simulink model "Powertrain_model_SEV_21b"  (R2021b)
settings: Solver=VariableStepAuto  StartTime=0.0  StopTime=tspan  RelTol=1e-3
values from neighbouring files (symbols this model uses):
  bsfc_idle_GE = 4.96e03    (= 4960)    [Sim_script.m]
  DR = 5.213    [Sim_script.m]
  drawn_pow_M = 464.6018    [Sim_script.m]
  Gensetdata = Gensetdata1    [Sim_script.m]
  motor_eff = motor_eff_PMSM    [Sim_script.m]
  Trans_In = 24.086    [Sim_script.m]
  tspan = 10800    [Sim_script.m]
  w_CE_idle = 400    [Sim_script.m]
undefined symbols (not defined in the file or in its folder): dailyloadl, eta_EM_map, resT_conv_bollard, resT_conv_free, resT_conv_tow, T_EM_col, T_EM_max, w_EM_row
libraries: slpidlib x1
settings Model: Creator=user  LastModifiedBy=olsonsao

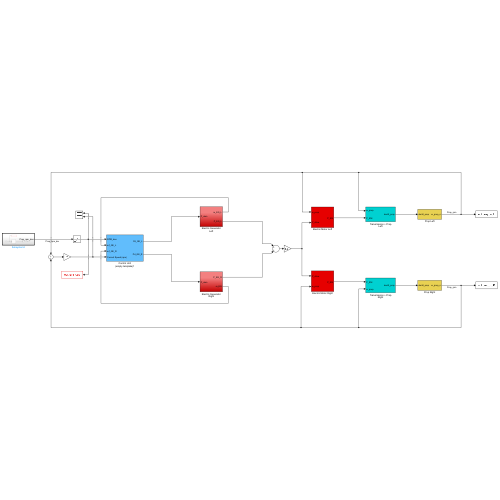
[thumbnail: Simulink's stored preview of the top-level diagram]
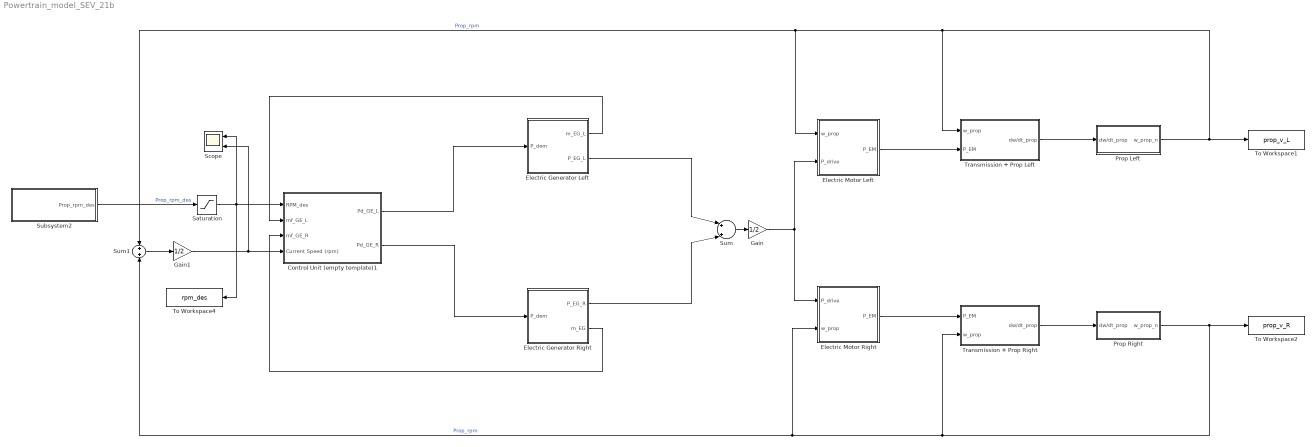
== system Powertrain_model_SEV_21b ==
  Control Unit (empty template)1 : Subsystem  Tag=control unit
  Electric Generator Left : Subsystem
  Electric Generator Right : Subsystem
  Electric Motor Left : Subsystem
  Electric Motor Right : Subsystem
  Gain : Gain  Gain=1/2
  Gain1 : Gain  Gain=1/2
  Prop Left : Subsystem
  Prop Right : Subsystem
  Saturation : Saturate  UpperLimit=inf  LowerLimit=w_CE_idle/DR
  Scope : Scope  NumInputPorts=2
  Subsystem2 : Subsystem  TreatAsAtomicUnit=on
  Sum : Sum  Inputs=|+|+|
  Sum1 : Sum  Inputs=+|+
  To Workspace1 : ToWorkspace  VariableName=prop_v_L  SampleTime=-1
      settings: Save2DSignal=2-D array (concatenate along first dimension)
  To Workspace2 : ToWorkspace  VariableName=prop_v_R  SampleTime=-1
      settings: Save2DSignal=2-D array (concatenate along first dimension)
  To Workspace4 : ToWorkspace  VariableName=rpm_des  SampleTime=-1
      settings: Save2DSignal=2-D array (concatenate along first dimension)
  Transmission + Prop Left : Subsystem
  Transmission + Prop Right : Subsystem
  wires:
  Sum/1 -> Gain/1
  Gain/1 -> Electric Motor Right/1(P_drive), Electric Motor Left/2(P_drive)
  Electric Motor Left/1(P_EM) -> Transmission + Prop Left/2(P_EM)
  Prop Left/1(w_prop_n) -> To Workspace1/1, Transmission + Prop Left/1(w_prop), Electric Motor Left/1(w_prop), Sum1/1  "Prop_rpm"
  Electric Motor Right/1(P_EM) -> Transmission + Prop Right/1(P_EM)
  Prop Right/1(w_prop_n) -> Transmission + Prop Right/2(w_prop), Electric Motor Right/2(w_prop), Sum1/2, To Workspace2/1  "Prop_rpm"
  Gain1/1 -> Scope/2, Control Unit (empty template)1/4(Current Speed (rpm))
  Subsystem2/1(Prop_rpm_des) -> Saturation/1  "Prop_rpm_des"
  Electric Generator Left/1(m_EG_L) -> Control Unit (empty template)1/2(mf_GE_L)
  Electric Generator Right/2(m_EG) -> Control Unit (empty template)1/3(mf_GE_R)
  Sum1/1 -> Gain1/1
  Transmission + Prop Left/1(dw/dt_prop) -> Prop Left/1(dw/dt_prop)
  Transmission + Prop Right/1(dw/dt_prop) -> Prop Right/1(dw/dt_prop)
  Control Unit (empty template)1/2(Pd_GE_R) -> Electric Generator Right/1(P_dem)
  Electric Generator Right/1(P_EG_R) -> Sum/2
  Control Unit (empty template)1/1(Pd_GE_L) -> Electric Generator Left/1(P_dem)
  Electric Generator Left/2(P_EG_L) -> Sum/1
  Saturation/1 -> Control Unit (empty template)1/1(RPM_des), To Workspace4/1, Scope/1

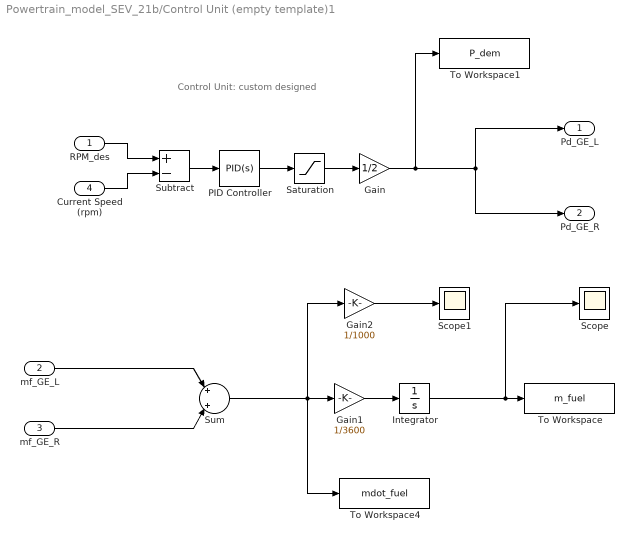
== system Powertrain_model_SEV_21b/Control Unit (empty template)1 ==
  note: Control Unit: custom designed
  RPM_des : Inport
  mf_GE_L : Inport  Port=2
  mf_GE_R : Inport  Port=3
  Current Speed (rpm) : Inport  Port=4
  Gain : Gain  Gain=1/2
  Gain1 : Gain  Gain=1/3600
  Gain2 : Gain  Gain=1/1000
  Integrator : Integrator
  PID Controller : slpidlib/PID Controller  Controller=PID  Form=Parallel  TimeDomain=Continuous-time  UseExternalTs=off  SampleTime=-1  IntegratorMethod=Forward Euler  FilterMethod=Forward Euler  ControllerParametersSource=internal  P=1.27731937948155  I=0.314602230470785  D=0.413734700213223  UseFilter=on  N=0.624884340967824  TunerSelectOption=Transfer Function Based (PID Tuner App)  InitialConditionSource=internal  InitialConditionForIntegrator=0  InitialConditionForFilter=0  DifferentiatorICPrevScaledInput=0  ExternalReset=none  TrackingMode=off  Kt=1  LimitOutput=on  SatLimitsSource=internal  UpperSaturationLimit=inf  LowerSaturationLimit=0  LinearizeAsGain=on  AntiWindupMode=none  Kb=1  POutMin=[]  POutMax=[]  IOutMin=[]  IOutMax=[]  DOutMin=[]  DOutMax=[]  NOutMin=[]  NOutMax=[]  SumOutMin=[]  SumOutMax=[]  SaturationOutMin=[]  SaturationOutMax=[]  PParamMin=[]  PParamMax=[]  IParamMin=[]  IParamMax=[]  DParamMin=[]  DParamMax=[]  NParamMin=[]  NParamMax=[]  KbParamMin=[]  KbParamMax=[]  KtParamMin=[]  KtParamMax=[]  KbOutMin=[]  KbOutMax=[]  KtOutMin=[]  KtOutMax=[]  IntegratorOutMin=[]  IntegratorOutMax=[]  FilterOutMin=[]  FilterOutMax=[]  SumI1OutMin=[]  SumI1OutMax=[]  SumI2OutMin=[]  SumI2OutMax=[]  SumI3OutMin=[]  SumI3OutMax=[]  SumI4OutMin=[]  SumI4OutMax=[]  SumDOutMin=[]  SumDOutMax=[]  DifferentiatorOutMin=[]  DifferentiatorOutMax=[]  FilterDiffOutCoefMin=[]  FilterDiffOutCoefMax=[]  ReciprocalOutMin=[]  ReciprocalOutMax=[]  SumDenOutMin=[]  SumDenOutMax=[]  SumNumOutMin=[]  SumNumOutMax=[]  DivideOutMin=[]  DivideOutMax=[]  UdiffTsProdOutMin=[]  UdiffTsProdOutMax=[]  NTsProdOutMin=[]  NTsProdOutMax=[]  UintegralTsProdOutMin=[]  UintegralTsProdOutMax=[]  UngainTsProdOutMin=[]  UngainTsProdOutMax=[]  IntegratorContinuousStateAttributes=''  IntegratorStateMustResolveToSignalObject=off  IntegratorRTWStateStorageClass=Auto  FilterContinuousStateAttributes=''  FilterStateMustResolveToSignalObject=off  FilterRTWStateStorageClass=Auto  ParallelPVariant=InternalParameters  IdealPVariant=Disabled  IVariant=InternalParameters  DVariant=InternalParameters  IntegratorVariant=Continuous  SatVariant=Enabled  AWVariant=Passthrough  PCopyVariant=Disabled  TRVariant=Disabled  FdbkBlocksVariant=Forward  IdealPFdbkVariant=Disabled  SatFdbkVariant=Disabled  DerivativeFilterVariant=ContFilter  NVariant=InternalParameters  NCopyVariant=Disabled  FilterICVariant=InternalICsFilter  IntegratorICVariant=InternalICs  ExternalResetVariant=Disabled  TRSumVariant=Passthrough  SumFdbkVariant=Disabled  SumVariant=Sum_PID  TsampFilterVariant=InternalTs  TsampNgainVariant=Passthrough  TsampIntegralVariant=Passthrough  ExternalSaturationOutDataTypeStr=Inherit: Same as second input
  Saturation : Saturate  UpperLimit=inf  LowerLimit=0
  Scope : Scope
  Scope1 : Scope
  Subtract : Sum  Inputs=+-
  Sum : Sum  Inputs=|+|+|
  To Workspace : ToWorkspace  VariableName=m_fuel  SampleTime=-1
      settings: Save2DSignal=2-D array (concatenate along first dimension)
  To Workspace1 : ToWorkspace  VariableName=P_dem  SampleTime=-1
      settings: Save2DSignal=2-D array (concatenate along first dimension)
  To Workspace4 : ToWorkspace  VariableName=mdot_fuel  SampleTime=-1
      settings: Save2DSignal=2-D array (concatenate along first dimension)
  Pd_GE_L : Outport  InitialOutput=0
  Pd_GE_R : Outport  Port=2  InitialOutput=0
  wires:
  Current Speed (rpm)/1 -> Subtract/2
  RPM_des/1 -> Subtract/1
  Subtract/1 -> PID Controller/1
  mf_GE_L/1 -> Sum/1
  mf_GE_R/1 -> Sum/2
  PID Controller/1 -> Saturation/1
  Saturation/1 -> Gain/1
  Gain/1 -> To Workspace1/1, Pd_GE_R/1, Pd_GE_L/1
  Gain1/1 -> Integrator/1
  Integrator/1 -> To Workspace/1, Scope/1
  Gain2/1 -> Scope1/1
  Sum/1 -> To Workspace4/1, Gain2/1, Gain1/1

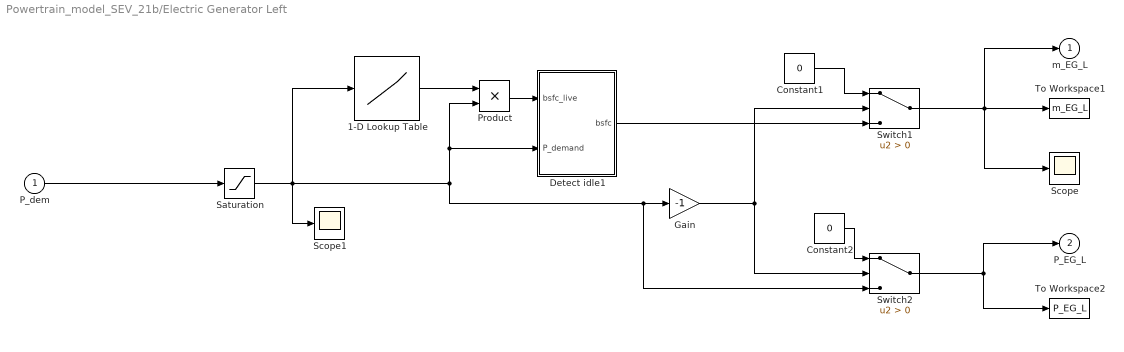
== system Powertrain_model_SEV_21b/Electric Generator Left ==
  P_dem : Inport
  1-D Lookup Table : Lookup_n-D  NumberOfTableDimensions=1  BreakpointsForDimension1=Gensetdata.('Power(kW)')  Table=Gensetdata.('Bsfc(g/kWh)')  InterpMethod=Cubic spline  ExtrapMethod=Cubic spline  InternalRulePriority=Speed  RndMeth=Simplest  InputSameDT=on
  Constant1 : Constant  Value=0
  Constant2 : Constant  Value=0
  Detect idle1 : Subsystem
  Gain : Gain  Gain=-1
  Product : Product
  Saturation : Saturate  UpperLimit=2500  LowerLimit=0
  Scope : Scope
  Scope1 : Scope
  Switch1 : Switch  Criteria=u2 > Threshold
  Switch2 : Switch  Criteria=u2 > Threshold
  To Workspace1 : ToWorkspace  VariableName=m_EG_L  SampleTime=-1
      settings: Save2DSignal=2-D array (concatenate along first dimension)
  To Workspace2 : ToWorkspace  VariableName=P_EG_L  SampleTime=-1
      settings: Save2DSignal=2-D array (concatenate along first dimension)
  m_EG_L : Outport  InitialOutput=0
  P_EG_L : Outport  Port=2  InitialOutput=0
  wires:
  1-D Lookup Table/1 -> Product/1
  Saturation/1 -> Scope1/1, Switch2/3, Gain/1, Detect idle1/2(P_demand), Product/2, 1-D Lookup Table/1
  P_dem/1 -> Saturation/1
  Product/1 -> Detect idle1/1(bsfc_live)
  Gain/1 -> Switch1/2, Switch2/2
  Constant1/1 -> Switch1/1
  Constant2/1 -> Switch2/1
  Detect idle1/1(bsfc) -> Switch1/3
  Switch1/1 -> Scope/1, To Workspace1/1, m_EG_L/1
  Switch2/1 -> To Workspace2/1, P_EG_L/1

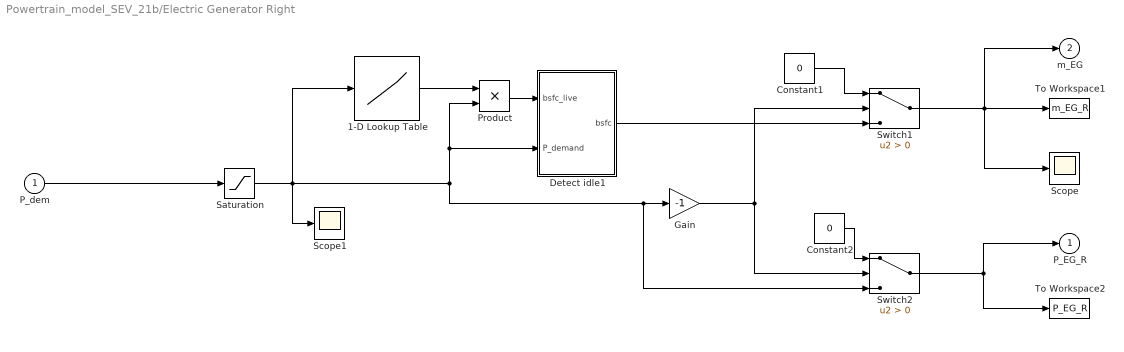
== system Powertrain_model_SEV_21b/Electric Generator Right ==
  P_dem : Inport
  1-D Lookup Table : Lookup_n-D  NumberOfTableDimensions=1  BreakpointsForDimension1=Gensetdata.('Power(kW)')  Table=Gensetdata.('Bsfc(g/kWh)')  InterpMethod=Cubic spline  ExtrapMethod=Cubic spline  InternalRulePriority=Speed  RndMeth=Simplest  InputSameDT=on
  Constant1 : Constant  Value=0
  Constant2 : Constant  Value=0
  Detect idle1 : Subsystem
  Gain : Gain  Gain=-1
  Product : Product
  Saturation : Saturate  UpperLimit=2500  LowerLimit=0
  Scope : Scope
  Scope1 : Scope
  Switch1 : Switch  Criteria=u2 > Threshold
  Switch2 : Switch  Criteria=u2 > Threshold
  To Workspace1 : ToWorkspace  VariableName=m_EG_R  SampleTime=-1
      settings: Save2DSignal=2-D array (concatenate along first dimension)
  To Workspace2 : ToWorkspace  VariableName=P_EG_R  SampleTime=-1
      settings: Save2DSignal=2-D array (concatenate along first dimension)
  P_EG_R : Outport  InitialOutput=0
  m_EG : Outport  Port=2  InitialOutput=0
  wires:
  1-D Lookup Table/1 -> Product/1
  Saturation/1 -> Scope1/1, Switch2/3, Gain/1, Detect idle1/2(P_demand), Product/2, 1-D Lookup Table/1
  P_dem/1 -> Saturation/1
  Product/1 -> Detect idle1/1(bsfc_live)
  Gain/1 -> Switch1/2, Switch2/2
  Constant1/1 -> Switch1/1
  Constant2/1 -> Switch2/1
  Detect idle1/1(bsfc) -> Switch1/3
  Switch1/1 -> Scope/1, To Workspace1/1, m_EG/1
  Switch2/1 -> To Workspace2/1, P_EG_R/1

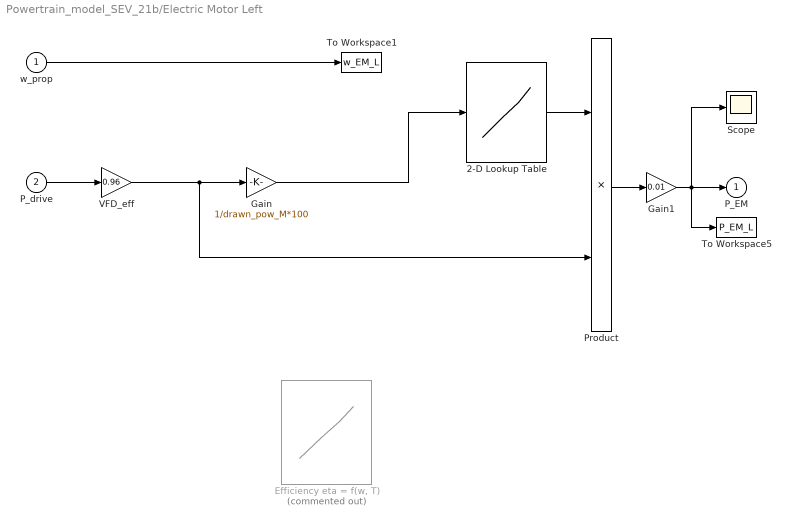
== system Powertrain_model_SEV_21b/Electric Motor Left ==
  w_prop : Inport
  P_drive : Inport  Port=2
  2-D Lookup Table : Lookup_n-D  NumberOfTableDimensions=1  BreakpointsForDimension1=motor_eff.('%power')  BreakpointsForDimension2=T_EM_col  Table=motor_eff.('eff')  InterpMethod=Cubic spline  ExtrapMethod=Cubic spline  InternalRulePriority=Speed  RndMeth=Simplest  InputSameDT=on
  "Efficiency eta = f(w, T)" : Lookup2D  Commented=on  RowIndex=w_EM_row  ColumnIndex=T_EM_col  Table=eta_EM_map
  Gain : Gain  Gain=1/drawn_pow_M*100
  Gain1 : Gain  Gain=0.01
  Product : Product  InputSameDT=on  RndMeth=Zero  SaturateOnIntegerOverflow=on  OutDataTypeStr=Inherit: Same as first input
  Scope : Scope
  To Workspace1 : ToWorkspace  VariableName=w_EM_L  SampleTime=-1
      settings: Save2DSignal=2-D array (concatenate along first dimension)
  To Workspace5 : ToWorkspace  VariableName=P_EM_L  SampleTime=-1
      settings: Save2DSignal=2-D array (concatenate along first dimension)
  VFD_eff : Gain  Gain=0.96
  P_EM : Outport  InitialOutput=0
  wires:
  Product/1 -> Gain1/1
  P_drive/1 -> VFD_eff/1
  2-D Lookup Table/1 -> Product/1
  w_prop/1 -> To Workspace1/1
  Gain/1 -> 2-D Lookup Table/1
  VFD_eff/1 -> Gain/1, Product/2
  Gain1/1 -> Scope/1, To Workspace5/1, P_EM/1

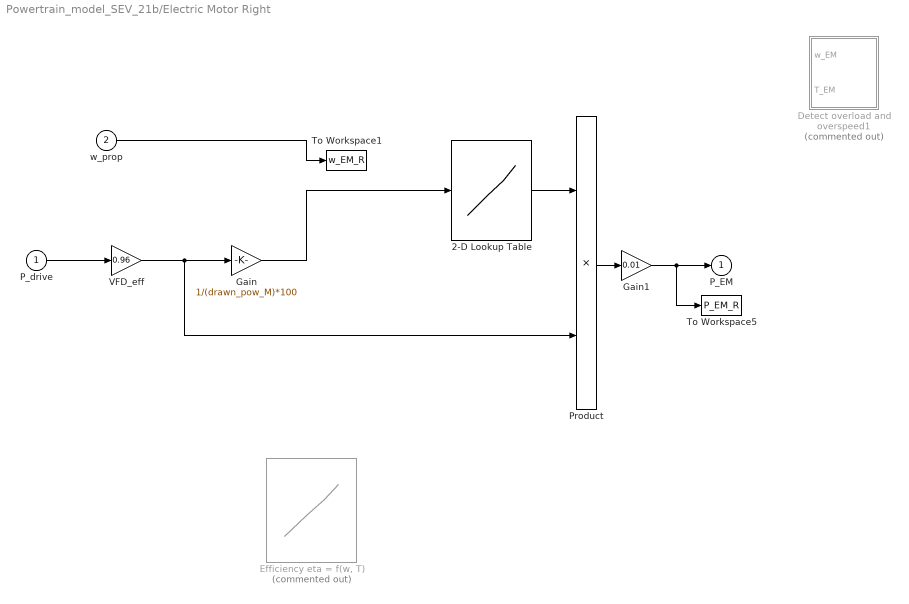
== system Powertrain_model_SEV_21b/Electric Motor Right ==
  P_drive : Inport
  w_prop : Inport  Port=2
  2-D Lookup Table : Lookup_n-D  NumberOfTableDimensions=1  BreakpointsForDimension1=motor_eff.('%power')  BreakpointsForDimension2=T_EM_col  Table=motor_eff.('eff')  InterpMethod=Cubic spline  ExtrapMethod=Cubic spline  InternalRulePriority=Speed  RndMeth=Simplest  InputSameDT=on
  Detect overload and overspeed1 : Subsystem  Commented=on
  "Efficiency eta = f(w, T)" : Lookup2D  Commented=on  RowIndex=w_EM_row  ColumnIndex=T_EM_col  Table=eta_EM_map
  Gain : Gain  Gain=1/(drawn_pow_M)*100
  Gain1 : Gain  Gain=0.01
  Product : Product  InputSameDT=on  RndMeth=Zero  SaturateOnIntegerOverflow=on  OutDataTypeStr=Inherit: Same as first input
  To Workspace1 : ToWorkspace  VariableName=w_EM_R  SampleTime=-1
      settings: Save2DSignal=2-D array (concatenate along first dimension)
  To Workspace5 : ToWorkspace  VariableName=P_EM_R  SampleTime=-1
      settings: Save2DSignal=2-D array (concatenate along first dimension)
  VFD_eff : Gain  Gain=0.96
  P_EM : Outport  InitialOutput=0
  wires:
  Product/1 -> Gain1/1
  P_drive/1 -> VFD_eff/1
  2-D Lookup Table/1 -> Product/1
  w_prop/1 -> To Workspace1/1
  Gain/1 -> 2-D Lookup Table/1
  VFD_eff/1 -> Gain/1, Product/2
  Gain1/1 -> To Workspace5/1, P_EM/1

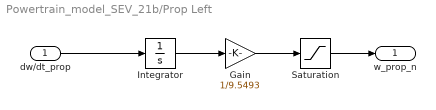
== system Powertrain_model_SEV_21b/Prop Left ==
  dw/dt_prop : Inport
  Gain : Gain  Gain=1/9.5493
  Integrator : Integrator  InitialCondition=w_CE_idle/DR  LowerSaturationLimit=1
  Saturation : Saturate  UpperLimit=inf  LowerLimit=0
  w_prop_n : Outport
  wires:
  dw/dt_prop/1 -> Integrator/1
  Integrator/1 -> Gain/1
  Saturation/1 -> w_prop_n/1
  Gain/1 -> Saturation/1

== system Powertrain_model_SEV_21b/Prop Right ==
  dw/dt_prop : Inport
  Gain : Gain  Gain=1/9.5493
  Integrator : Integrator  InitialCondition=w_CE_idle/DR  LowerSaturationLimit=1
  Saturation : Saturate  UpperLimit=inf  LowerLimit=0
  w_prop_n : Outport
  wires:
  dw/dt_prop/1 -> Integrator/1
  Integrator/1 -> Gain/1
  Saturation/1 -> w_prop_n/1
  Gain/1 -> Saturation/1

== system Powertrain_model_SEV_21b/Subsystem2 ==
  1-D Lookup Table : Lookup_n-D  NumberOfTableDimensions=1  BreakpointsForDimension1=[1:10800]  Table=dailyloadl.('m_sec')  InternalRulePriority=Speed  RndMeth=Simplest  InputSameDT=on
  Clock : Clock
  Gain : Gain
  To Workspace3 : ToWorkspace  VariableName=t  SampleTime=-1
      settings: Save2DSignal=2-D array (concatenate along first dimension)
  Prop_rpm_des : Outport
  wires:
  Clock/1 -> To Workspace3/1, 1-D Lookup Table/1
  1-D Lookup Table/1 -> Gain/1
  Gain/1 -> Prop_rpm_des/1

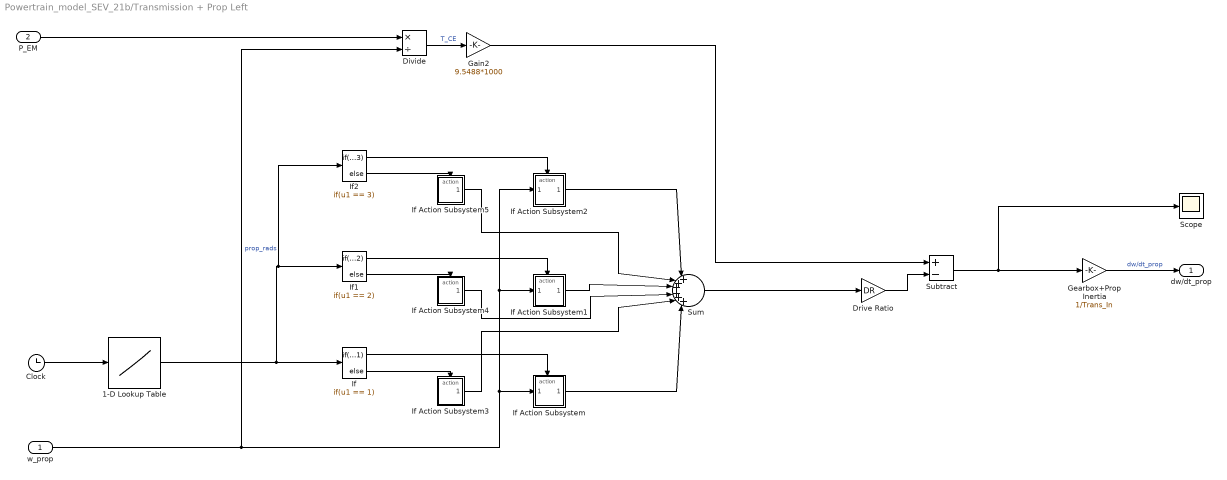
== system Powertrain_model_SEV_21b/Transmission + Prop Left ==
  w_prop : Inport
  P_EM : Inport  Port=2
  1-D Lookup Table : Lookup_n-D  NumberOfTableDimensions=1  BreakpointsForDimension1=[1:tspan]  Table=dailyloadl.('m_mode')  InternalRulePriority=Speed  RndMeth=Simplest  InputSameDT=on
  Clock : Clock
  Divide : Product  Inputs=*/
  Drive Ratio : Gain  Gain=DR
  Gain2 : Gain  Gain=9.5488*1000
  Gearbox+Prop Inertia : Gain  Gain=1/Trans_In
  If : If  IfExpression=u1 == 1
  If Action Subsystem : Subsystem  TreatAsAtomicUnit=on
  If Action Subsystem1 : Subsystem  TreatAsAtomicUnit=on
  If Action Subsystem2 : Subsystem  TreatAsAtomicUnit=on
  If Action Subsystem3 : Subsystem  TreatAsAtomicUnit=on
  If Action Subsystem4 : Subsystem  TreatAsAtomicUnit=on
  If Action Subsystem5 : Subsystem  TreatAsAtomicUnit=on
  If1 : If  IfExpression=u1 == 2
  If2 : If  IfExpression=u1 == 3
  Scope : Scope
  Subtract : Sum  Inputs=+-
  Sum : Sum  Inputs=|++++++|
  dw/dt_prop : Outport
  wires:
  P_EM/1 -> Divide/1
  Gearbox+Prop Inertia/1 -> dw/dt_prop/1  "dw/dt_prop"
  Subtract/1 -> Gearbox+Prop Inertia/1, Scope/1
  Divide/1 -> Gain2/1  "T_CE"
  Gain2/1 -> Subtract/1
  w_prop/1 -> If Action Subsystem2/1(w_prop), If Action Subsystem1/1(w_prop), If Action Subsystem/1(w_prop), Divide/2  "prop_rads"
  Drive Ratio/1 -> Subtract/2
  1-D Lookup Table/1 -> If2/1, If1/1, If/1
  Clock/1 -> 1-D Lookup Table/1
  If/1 -> If Action Subsystem/Action
  If/2 -> If Action Subsystem3/Action
  If1/1 -> If Action Subsystem1/Action
  If2/1 -> If Action Subsystem2/Action
  If2/2 -> If Action Subsystem5/Action
  If1/2 -> If Action Subsystem4/Action
  If Action Subsystem2/1(Out1) -> Sum/1
  If Action Subsystem5/1(Out1) -> Sum/2
  If Action Subsystem/1(Out1) -> Sum/6
  If Action Subsystem3/1(Out1) -> Sum/5
  If Action Subsystem1/1(Out1) -> Sum/3
  If Action Subsystem4/1(Out1) -> Sum/4
  Sum/1 -> Drive Ratio/1

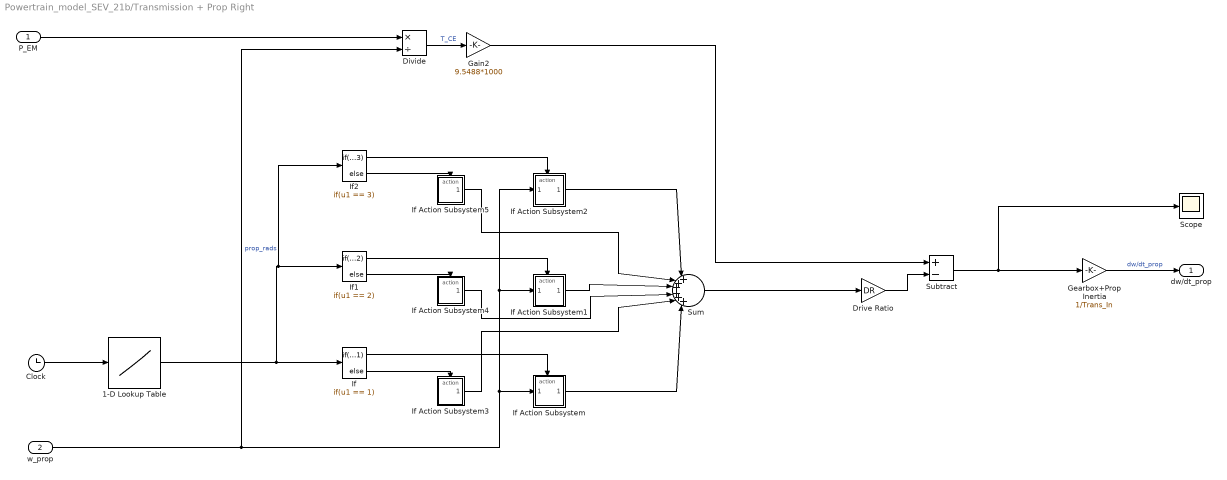
== system Powertrain_model_SEV_21b/Transmission + Prop Right ==
  P_EM : Inport
  w_prop : Inport  Port=2
  1-D Lookup Table : Lookup_n-D  NumberOfTableDimensions=1  BreakpointsForDimension1=[1:tspan]  Table=dailyloadl.('m_mode')  InternalRulePriority=Speed  RndMeth=Simplest  InputSameDT=on
  Clock : Clock
  Divide : Product  Inputs=*/
  Drive Ratio : Gain  Gain=DR
  Gain2 : Gain  Gain=9.5488*1000
  Gearbox+Prop Inertia : Gain  Gain=1/Trans_In
  If : If  IfExpression=u1 == 1
  If Action Subsystem : Subsystem  TreatAsAtomicUnit=on
  If Action Subsystem1 : Subsystem  TreatAsAtomicUnit=on
  If Action Subsystem2 : Subsystem  TreatAsAtomicUnit=on
  If Action Subsystem3 : Subsystem  TreatAsAtomicUnit=on
  If Action Subsystem4 : Subsystem  TreatAsAtomicUnit=on
  If Action Subsystem5 : Subsystem  TreatAsAtomicUnit=on
  If1 : If  IfExpression=u1 == 2
  If2 : If  IfExpression=u1 == 3
  Scope : Scope
  Subtract : Sum  Inputs=+-
  Sum : Sum  Inputs=|++++++|
  dw/dt_prop : Outport
  wires:
  P_EM/1 -> Divide/1
  Gearbox+Prop Inertia/1 -> dw/dt_prop/1  "dw/dt_prop"
  Subtract/1 -> Gearbox+Prop Inertia/1, Scope/1
  Divide/1 -> Gain2/1  "T_CE"
  Gain2/1 -> Subtract/1
  w_prop/1 -> If Action Subsystem2/1(w_prop), If Action Subsystem1/1(w_prop), If Action Subsystem/1(w_prop), Divide/2  "prop_rads"
  Drive Ratio/1 -> Subtract/2
  1-D Lookup Table/1 -> If2/1, If1/1, If/1
  Clock/1 -> 1-D Lookup Table/1
  If/1 -> If Action Subsystem/Action
  If/2 -> If Action Subsystem3/Action
  If1/1 -> If Action Subsystem1/Action
  If2/1 -> If Action Subsystem2/Action
  If2/2 -> If Action Subsystem5/Action
  If1/2 -> If Action Subsystem4/Action
  If Action Subsystem2/1(Out1) -> Sum/1
  If Action Subsystem5/1(Out1) -> Sum/2
  If Action Subsystem/1(Out1) -> Sum/6
  If Action Subsystem3/1(Out1) -> Sum/5
  If Action Subsystem1/1(Out1) -> Sum/3
  If Action Subsystem4/1(Out1) -> Sum/4
  Sum/1 -> Drive Ratio/1

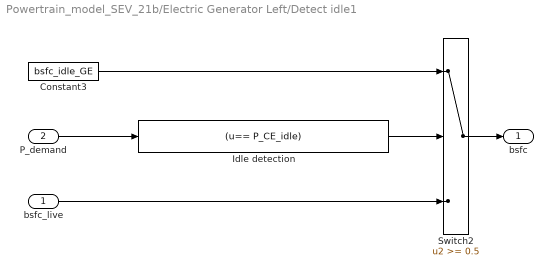
== system Powertrain_model_SEV_21b/Electric Generator Left/Detect idle1 ==
  bsfc_live : Inport
  P_demand : Inport  Port=2
  Constant3 : Constant  Value=bsfc_idle_GE
  Idle detection : Fcn  Expr=(u== P_CE_idle)
  Switch2 : Switch  Threshold=0.5  SaturateOnIntegerOverflow=on  InputSameDT=on
  bsfc : Outport  InitialOutput=0
  wires:
  P_demand/1 -> Idle detection/1
  Idle detection/1 -> Switch2/2
  bsfc_live/1 -> Switch2/3
  Switch2/1 -> bsfc/1
  Constant3/1 -> Switch2/1

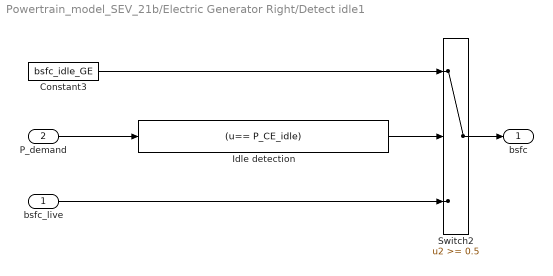
== system Powertrain_model_SEV_21b/Electric Generator Right/Detect idle1 ==
  bsfc_live : Inport
  P_demand : Inport  Port=2
  Constant3 : Constant  Value=bsfc_idle_GE
  Idle detection : Fcn  Expr=(u== P_CE_idle)
  Switch2 : Switch  Threshold=0.5  SaturateOnIntegerOverflow=on  InputSameDT=on
  bsfc : Outport  InitialOutput=0
  wires:
  P_demand/1 -> Idle detection/1
  Idle detection/1 -> Switch2/2
  bsfc_live/1 -> Switch2/3
  Switch2/1 -> bsfc/1
  Constant3/1 -> Switch2/1

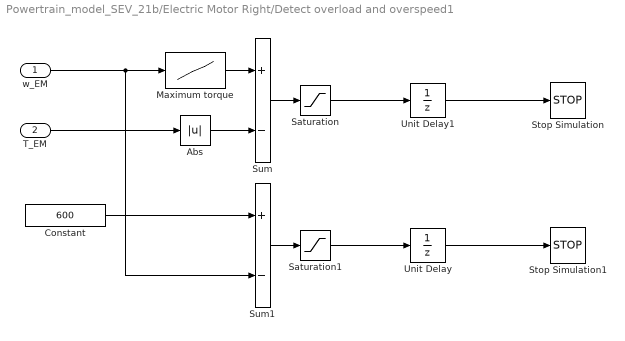
== system Powertrain_model_SEV_21b/Electric Motor Right/Detect overload and overspeed1 ==
  w_EM : Inport
  T_EM : Inport  Port=2
  Abs : Abs  SaturateOnIntegerOverflow=on
  Constant : Constant  Value=600
  Maximum torque : Lookup  InputValues=w_EM_row  Table=T_EM_max  SaturateOnIntegerOverflow=on
  Saturation : Saturate  UpperLimit=0  LowerLimit=-inf
  Saturation1 : Saturate  UpperLimit=0  LowerLimit=-inf
  Stop Simulation : Stop
  Stop Simulation1 : Stop
  Sum : Sum  Inputs=+-  InputSameDT=on  SaturateOnIntegerOverflow=on  OutDataTypeStr=Inherit: Same as first input
  Sum1 : Sum  Inputs=+-  InputSameDT=on  SaturateOnIntegerOverflow=on  OutDataTypeStr=Inherit: Same as first input
  Unit Delay : UnitDelay  SampleTime=-1  HasFrameUpgradeWarning=on
  Unit Delay1 : UnitDelay  SampleTime=-1  HasFrameUpgradeWarning=on
  wires:
  Saturation1/1 -> Unit Delay/1
  Sum1/1 -> Saturation1/1
  Constant/1 -> Sum1/1
  Saturation/1 -> Unit Delay1/1
  Abs/1 -> Sum/2
  Maximum torque/1 -> Sum/1
  T_EM/1 -> Abs/1
  w_EM/1 -> Sum1/2, Maximum torque/1
  Sum/1 -> Saturation/1
  Unit Delay/1 -> Stop Simulation1/1
  Unit Delay1/1 -> Stop Simulation/1

== system Powertrain_model_SEV_21b/Transmission + Prop Left/If Action Subsystem ==
  w_prop : Inport
  Action Port : ActionPort  ActionPortLabel=if(u1 == 1)
  Gain : Gain  Gain=DR
  Lookup with Linear Point-slope Interpolation1 : Lookup_n-D  NumberOfTableDimensions=1  BreakpointsForDimension1=resT_conv_free.('rpm')  Table=resT_conv_free.('resT')  InternalRulePriority=Speed  RndMeth=Simplest  InputSameDT=on
  Out1 : Outport
  wires:
  Lookup with Linear Point-slope Interpolation1/1 -> Out1/1
  w_prop/1 -> Gain/1  "prop_rads"
  Gain/1 -> Lookup with Linear Point-slope Interpolation1/1

== system Powertrain_model_SEV_21b/Transmission + Prop Left/If Action Subsystem1 ==
  w_prop : Inport
  Action Port : ActionPort  ActionPortLabel=if(u1 == 1)
  Gain1 : Gain  Gain=DR
  Lookup with Linear Point-slope Interpolation2 : Lookup_n-D  NumberOfTableDimensions=1  BreakpointsForDimension1=resT_conv_tow.('rpm')  Table=resT_conv_tow.('resT')  InternalRulePriority=Speed  RndMeth=Simplest  InputSameDT=on
  Out1 : Outport
  wires:
  Lookup with Linear Point-slope Interpolation2/1 -> Out1/1
  Gain1/1 -> Lookup with Linear Point-slope Interpolation2/1
  w_prop/1 -> Gain1/1  "prop_rads"

== system Powertrain_model_SEV_21b/Transmission + Prop Left/If Action Subsystem2 ==
  w_prop : Inport
  Action Port : ActionPort  ActionPortLabel=if(u1 == 1)
  Gain3 : Gain  Gain=DR
  Lookup with Linear Point-slope Interpolation3 : Lookup_n-D  NumberOfTableDimensions=1  BreakpointsForDimension1=resT_conv_bollard.('rpm')  Table=resT_conv_bollard.('resT')  InternalRulePriority=Speed  RndMeth=Simplest  InputSameDT=on
  Out1 : Outport
  wires:
  Lookup with Linear Point-slope Interpolation3/1 -> Out1/1
  Gain3/1 -> Lookup with Linear Point-slope Interpolation3/1
  w_prop/1 -> Gain3/1  "prop_rads"

== system Powertrain_model_SEV_21b/Transmission + Prop Left/If Action Subsystem3 ==
  Action Port : ActionPort  ActionPortLabel=else
  Constant : Constant  Value=0
  Out1 : Outport
  wires:
  Constant/1 -> Out1/1

== system Powertrain_model_SEV_21b/Transmission + Prop Left/If Action Subsystem4 ==
  Action Port : ActionPort  ActionPortLabel=else
  Constant : Constant  Value=0
  Out1 : Outport
  wires:
  Constant/1 -> Out1/1

== system Powertrain_model_SEV_21b/Transmission + Prop Left/If Action Subsystem5 ==
  Action Port : ActionPort  ActionPortLabel=else
  Constant : Constant  Value=0
  Out1 : Outport
  wires:
  Constant/1 -> Out1/1

== system Powertrain_model_SEV_21b/Transmission + Prop Right/If Action Subsystem ==
  w_prop : Inport
  Action Port : ActionPort
  Gain : Gain  Gain=DR
  Lookup with Linear Point-slope Interpolation1 : Lookup_n-D  NumberOfTableDimensions=1  BreakpointsForDimension1=resT_conv_free.('rpm')  Table=resT_conv_free.('resT')  InternalRulePriority=Speed  RndMeth=Simplest  InputSameDT=on
  Out1 : Outport
  wires:
  Lookup with Linear Point-slope Interpolation1/1 -> Out1/1
  w_prop/1 -> Gain/1  "prop_rads"
  Gain/1 -> Lookup with Linear Point-slope Interpolation1/1

== system Powertrain_model_SEV_21b/Transmission + Prop Right/If Action Subsystem1 ==
  w_prop : Inport
  Action Port : ActionPort
  Gain1 : Gain  Gain=DR
  Lookup with Linear Point-slope Interpolation2 : Lookup_n-D  NumberOfTableDimensions=1  BreakpointsForDimension1=resT_conv_tow.('rpm')  Table=resT_conv_tow.('resT')  InternalRulePriority=Speed  RndMeth=Simplest  InputSameDT=on
  Out1 : Outport
  wires:
  Lookup with Linear Point-slope Interpolation2/1 -> Out1/1
  Gain1/1 -> Lookup with Linear Point-slope Interpolation2/1
  w_prop/1 -> Gain1/1  "prop_rads"

== system Powertrain_model_SEV_21b/Transmission + Prop Right/If Action Subsystem2 ==
  w_prop : Inport
  Action Port : ActionPort
  Gain3 : Gain  Gain=DR
  Lookup with Linear Point-slope Interpolation3 : Lookup_n-D  NumberOfTableDimensions=1  BreakpointsForDimension1=resT_conv_bollard.('rpm')  Table=resT_conv_bollard.('resT')  InternalRulePriority=Speed  RndMeth=Simplest  InputSameDT=on
  Out1 : Outport
  wires:
  Lookup with Linear Point-slope Interpolation3/1 -> Out1/1
  Gain3/1 -> Lookup with Linear Point-slope Interpolation3/1
  w_prop/1 -> Gain3/1  "prop_rads"

== system Powertrain_model_SEV_21b/Transmission + Prop Right/If Action Subsystem3 ==
  Action Port : ActionPort
  Constant : Constant  Value=0
  Out1 : Outport
  wires:
  Constant/1 -> Out1/1

== system Powertrain_model_SEV_21b/Transmission + Prop Right/If Action Subsystem4 ==
  Action Port : ActionPort
  Constant : Constant  Value=0
  Out1 : Outport
  wires:
  Constant/1 -> Out1/1

== system Powertrain_model_SEV_21b/Transmission + Prop Right/If Action Subsystem5 ==
  Action Port : ActionPort
  Constant : Constant  Value=0
  Out1 : Outport
  wires:
  Constant/1 -> Out1/1
